simulink library "Scope_new"  (R2017b)
settings: Solver=VariableStepAuto  StartTime=0.0  StopTime=10.0  RelTol=1e-3
undefined symbols (not defined in the file): cal, CycLength, CycNmb, Engine, ess, gb, StopIndex
libraries: simulink x8, EC2_libraries x2
settings Model: Creator=Lyu19  LastModifiedBy=Lyu19

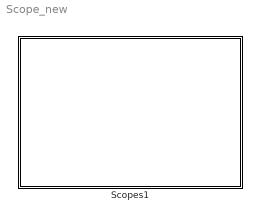
== system Scope_new ==
  Scopes1 : Subsystem
      mask Display: image('Images/Scope.jpg')

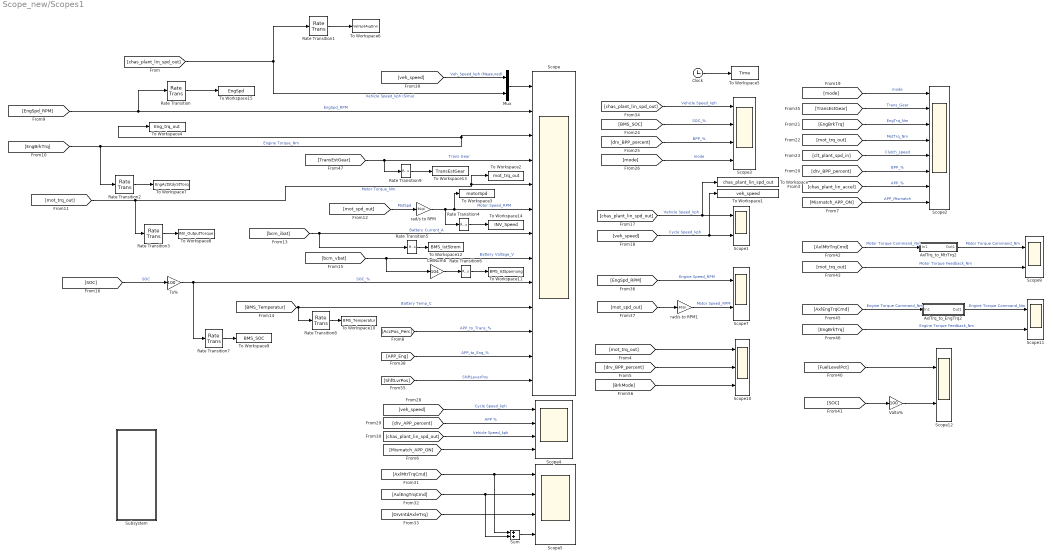
== system Scope_new/Scopes1 ==
  AxlTrq_to_EngTrq2 : Subsystem
  AxlTrq_to_MtrTrq2 : Subsystem
  CellNumb : Gain  Gain=104
  Clock : Clock
      settings: Decimation=WORKSPACE_DECIMATION
  Mux : Mux  Inputs=2
  Rate Transition{,1..9} (10 alike) : RateTransition  OutPortSampleTime=1
  Scope : Scope  NumInputPorts=13
  Scope{1,7,9,11..12} (5 alike) : Scope  NumInputPorts=2
  Scope10 : Scope  NumInputPorts=3
  Scope2 : Scope  NumInputPorts=8
  Scope3 : Scope  NumInputPorts=4
  Scope4 : Scope  NumInputPorts=4
  Scope5 : Scope  NumInputPorts=4
  Subsystem : Subsystem
  Sum : Sum
  To Workspace : ToWorkspace  VariableName=chas_plant_lin_spd_out  SampleTime=-1
  To Workspace1 : ToWorkspace  VariableName=veh_speed  SampleTime=-1
  To Workspace10 : ToWorkspace  VariableName=BMS_Temperatur  SampleTime=-1
  To Workspace11 : ToWorkspace  VariableName=BMS_IstSpannung  SampleTime=-1
  To Workspace12 : ToWorkspace  VariableName=BMS_IstStrom  SampleTime=-1
  To Workspace13 : ToWorkspace  VariableName=TransEstGear  SampleTime=-1
  To Workspace14 : ToWorkspace  VariableName=INV_Speed  SampleTime=-1
  To Workspace15 : ToWorkspace  VariableName=EngSpd  SampleTime=-1
  To Workspace2 : ToWorkspace  VariableName=mot_trq_out  SampleTime=-1
  To Workspace3 : ToWorkspace  VariableName=motorSpd  SampleTime=-1
  To Workspace4 : ToWorkspace  VariableName=Eng_trq_out  SampleTime=-1
  To Workspace5 : ToWorkspace  VariableName=Time  SampleTime=-1
      settings: Decimation=WORKSPACE_DECIMATION
  To Workspace6 : ToWorkspace  VariableName=VehSpdAvgDrvn  SampleTime=-1
  To Workspace7 : ToWorkspace  VariableName=EngActStdyStTorq  SampleTime=-1
  To Workspace8 : ToWorkspace  VariableName=INV_OutputTorque  SampleTime=-1
  To Workspace9 : ToWorkspace  VariableName=BMS_SOC  SampleTime=-1
  To% : Gain  Gain=100
  Valto% : Gain  Gain=100
  rad/s to RPM : Gain  Gain=30/pi
  rad/s to RPM1 : Gain  Gain=30/pi
  wires:
  [chas_plant_lin_spd_out] -> Rate Transition1/1, Mux/2  "Vehicle Speed_kph (Simu)"
  [EngSpd_RPM] -> Rate Transition/1, Scope/2  "EngSpd_RPM"
  [EngBrkTrq] -> Rate Transition2/1, Scope/3, To Workspace4/1  "Engine Torque_Nm"
  [mot_spd_out] -> rad/s to RPM/1  "MotSpd"
  [BMS_Temperatur] -> Rate Transition8/1, Scope/10  "Battery Temp_C"
  rad/s to RPM/1 -> Rate Transition4/1, To Workspace3/1, Scope/6  "Motor Speed_RPM"
  [mot_trq_out] -> Rate Transition3/1, To Workspace2/1, Scope/5  "Motor Torque_Nm"
  To%/1 -> Rate Transition7/1, Scope/9  "SOC_%"
  [TransEstGear] -> Rate Transition9/1, Scope/4  "Trans Gear"
  [bcm_ibat] -> Rate Transition5/1, Scope/7  "Battery Current_A"
  [chas_plant_lin_spd_out] -> Scope3/1  "Vehicle Speed_kph"
  [BMS_SOC] -> Scope3/2  "SOC_%"
  [drv_BPP_percent] -> Scope3/3  "BPP_%"
  [mode] -> Scope3/4  "mode"
  [chas_plant_lin_spd_out] -> To Workspace/1, Scope1/1  "Vehicle Speed_kph"
  [veh_speed] -> To Workspace1/1, Scope1/2  "Cycle Speed_kph"
  [mode] -> Scope2/1  "mode"
  [EngBrkTrq] -> Scope2/3  "EngTrq_Nm"
  [mot_trq_out] -> Scope2/4  "MotTrq_Nm"
  [clt_plant_spd_in] -> Scope2/5  "Clutch_speed"
  [EngSpd_RPM] -> Scope7/1  "Engine Speed_RPM"
  [mot_spd_out] -> rad/s to RPM1/1
  rad/s to RPM1/1 -> Scope7/2  "Motor Speed_RPM"
  [veh_speed] -> Scope4/1  "Cycle Speed_kph"
  [drv_APP_percent] -> Scope4/2  "APP %"
  [chas_plant_lin_spd_out] -> Scope4/3  "Vehicle Speed_kph"
  [AxlMtrTrqCmd] -> Sum/1, Scope5/1
  [AxlEngTrqCmd] -> Sum/2, Scope5/2
  [DrvIntdAxleTrq] -> Scope5/3
  Sum/1 -> Scope5/4
  [AxlMtrTrqCmd] -> AxlTrq_to_MtrTrq2/1(In1)  "Motor Torque Command_Nm"
  [mot_trq_out] -> Scope9/2  "Motor Torque Feedback_Nm"
  [AxlEngTrqCmd] -> AxlTrq_to_EngTrq2/1(In1)  "Engine Torque Command_Nm"
  [EngBrkTrq] -> Scope11/2  "Engine Torque Feedback_Nm"
  [TransEstGear] -> Scope2/2  "Trans_Gear"
  [drv_BPP_percent] -> Scope2/6  "BPP_%"
  [chas_plant_lin_accel] -> Scope2/7  "APP_%"
  AxlTrq_to_MtrTrq2/1(Out1) -> Scope9/1  "Motor Torque Command_Nm"
  AxlTrq_to_EngTrq2/1(Out1) -> Scope11/1  "Engine Torque Command_Nm"
  [bcm_vbat] -> Scope/8, CellNumb/1  "Battery Voltage_V"
  [Mismatch_APP_ON] -> Scope4/4
  [Mismatch_APP_ON] -> Scope2/8  "APP_Mismatch"
  [SOC] -> To%/1  "SOC"
  [AccPos_Perc] -> Scope/11  "APP_to_Trans_%"
  [APP_Eng] -> Scope/12  "APP_to_Eng_%"
  Mux/1 -> Scope/1
  [veh_speed] -> Mux/1  "Veh_Speed_kph (Measured)"
  Clock/1 -> To Workspace5/1
  [FuelLevelPct] -> Scope12/1
  [SOC] -> Valto%/1
  Valto%/1 -> Scope12/2
  [ShftLvrPos] -> Scope/13  "ShiftLeverPos"
  [mot_trq_out] -> Scope10/1
  [drv_BPP_percent] -> Scope10/2
  [BrkMode] -> Scope10/3
  CellNumb/1 -> Rate Transition6/1
  Rate Transition/1 -> To Workspace15/1
  Rate Transition1/1 -> To Workspace6/1
  Rate Transition2/1 -> To Workspace7/1
  Rate Transition3/1 -> To Workspace8/1
  Rate Transition4/1 -> To Workspace14/1
  Rate Transition5/1 -> To Workspace12/1
  Rate Transition6/1 -> To Workspace11/1
  Rate Transition7/1 -> To Workspace9/1
  Rate Transition8/1 -> To Workspace10/1
  Rate Transition9/1 -> To Workspace13/1

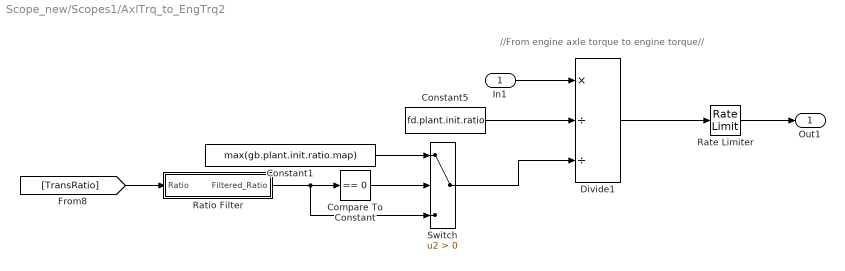
== system Scope_new/Scopes1/AxlTrq_to_EngTrq2 ==
  note: //From engine axle torque to engine torque//
  In1 : Inport
  Compare To Constant : simulink/Logic and Bit Operations/Compare To Constant  relop===  const=0  OutDataTypeStr=boolean
  Constant1 : Constant  Value=max(gb.plant.init.ratio.map)
  Constant5 : Constant  Value=fd.plant.init.ratio
  Divide1 : Product  Inputs=*//
  Rate Limiter : RateLimiter  RisingSlewLimit=Engine.trq_uprate  FallingSlewLimit=Engine.trq_derate
  Ratio Filter : Subsystem
  Switch : Switch  Criteria=u2 > Threshold
  Out1 : Outport
  wires:
  In1/1 -> Divide1/1
  Constant5/1 -> Divide1/2
  Divide1/1 -> Rate Limiter/1
  [TransRatio] -> Ratio Filter/1(Ratio)
  Compare To Constant/1 -> Switch/2
  Constant1/1 -> Switch/1
  Switch/1 -> Divide1/3
  Rate Limiter/1 -> Out1/1
  Ratio Filter/1(Filtered_Ratio) -> Switch/3, Compare To Constant/1

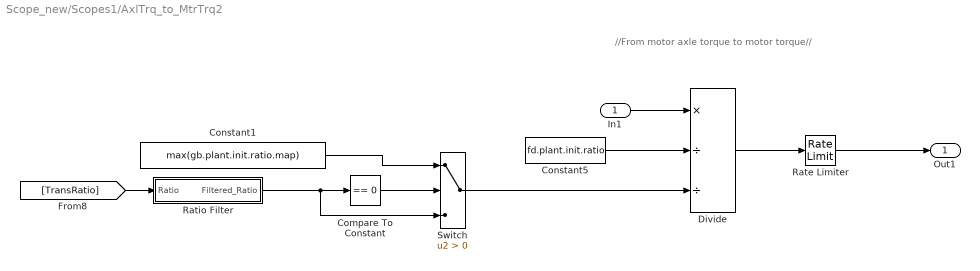
== system Scope_new/Scopes1/AxlTrq_to_MtrTrq2 ==
  note: //From motor axle torque to motor torque//
  In1 : Inport
  Compare To Constant : simulink/Logic and Bit Operations/Compare To Constant  relop===  const=0  OutDataTypeStr=boolean
  Constant1 : Constant  Value=max(gb.plant.init.ratio.map)
  Constant5 : Constant  Value=fd.plant.init.ratio
  Divide : Product  Inputs=*//
  Rate Limiter : RateLimiter  RisingSlewLimit=mcu.plant.init.trq_uprate  FallingSlewLimit=mcu.plant.init.trq_derate
  Ratio Filter : Subsystem
  Switch : Switch  Criteria=u2 > Threshold
  Out1 : Outport
  wires:
  In1/1 -> Divide/1
  Constant5/1 -> Divide/2
  Divide/1 -> Rate Limiter/1
  [TransRatio] -> Ratio Filter/1(Ratio)
  Compare To Constant/1 -> Switch/2
  Constant1/1 -> Switch/1
  Rate Limiter/1 -> Out1/1
  Switch/1 -> Divide/3
  Ratio Filter/1(Filtered_Ratio) -> Switch/3, Compare To Constant/1

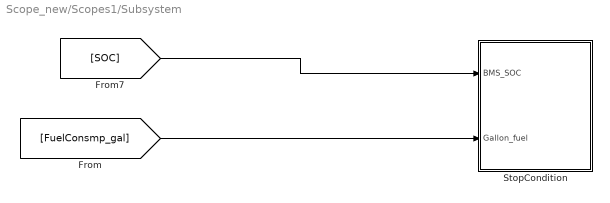
== system Scope_new/Scopes1/Subsystem ==
  "StopCondition " : Subsystem
  wires:
  [SOC] -> "StopCondition "/1(BMS_SOC)
  [FuelConsmp_gal] -> "StopCondition "/2(Gallon_fuel)

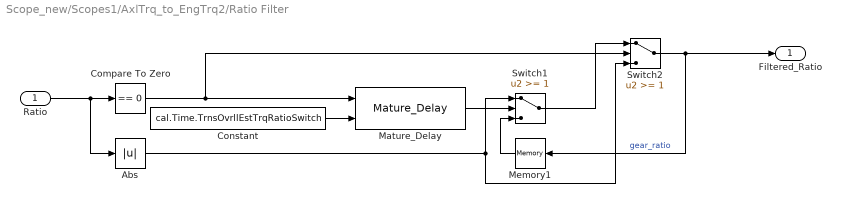
== system Scope_new/Scopes1/AxlTrq_to_EngTrq2/Ratio Filter ==
  Ratio : Inport
  Abs : Abs
  Compare To Zero : simulink/Logic and Bit Operations/Compare To Zero  relop===  OutDataTypeStr=boolean
  Constant : Constant  Value=cal.Time.TrnsOvrllEstTrqRatioSwitch
  Mature_Delay : EC2_libraries/Mature_Delay
      settings: SourceProductName=The database C:\Users\vrajm\AppData\Roaming\MathWorks\MATLAB\R2017b\slblocks_master.db is locked, or a table in the database is locked. (database is locked)
  Memory1 : Memory  InitialCondition=1
  Switch1 : Switch  Threshold=1
  Switch2 : Switch  Threshold=1
  Filtered_Ratio : Outport
  wires:
  Ratio/1 -> Compare To Zero/1, Abs/1
  Compare To Zero/1 -> Mature_Delay/1, Switch2/2
  Abs/1 -> Switch1/1, Switch2/3
  Switch1/1 -> Switch2/1
  Constant/1 -> Mature_Delay/2
  Mature_Delay/1 -> Switch1/2
  Memory1/1 -> Switch1/3
  Switch2/1 -> Filtered_Ratio/1, Memory1/1  "gear_ratio"

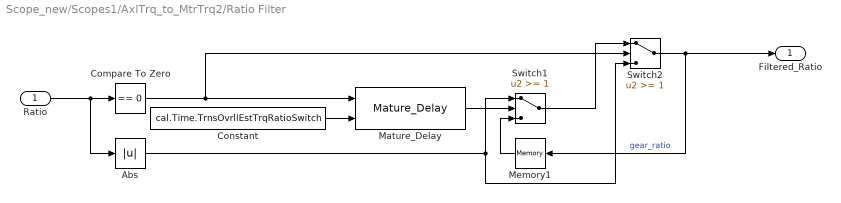
== system Scope_new/Scopes1/AxlTrq_to_MtrTrq2/Ratio Filter ==
  Ratio : Inport
  Abs : Abs
  Compare To Zero : simulink/Logic and Bit Operations/Compare To Zero  relop===  OutDataTypeStr=boolean
  Constant : Constant  Value=cal.Time.TrnsOvrllEstTrqRatioSwitch
  Mature_Delay : EC2_libraries/Mature_Delay
      settings: SourceProductName=The database C:\Users\vrajm\AppData\Roaming\MathWorks\MATLAB\R2017b\slblocks_master.db is locked, or a table in the database is locked. (database is locked)
  Memory1 : Memory  InitialCondition=1
  Switch1 : Switch  Threshold=1
  Switch2 : Switch  Threshold=1
  Filtered_Ratio : Outport
  wires:
  Ratio/1 -> Compare To Zero/1, Abs/1
  Compare To Zero/1 -> Mature_Delay/1, Switch2/2
  Abs/1 -> Switch1/1, Switch2/3
  Switch1/1 -> Switch2/1
  Constant/1 -> Mature_Delay/2
  Mature_Delay/1 -> Switch1/2
  Memory1/1 -> Switch1/3
  Switch2/1 -> Filtered_Ratio/1, Memory1/1  "gear_ratio"

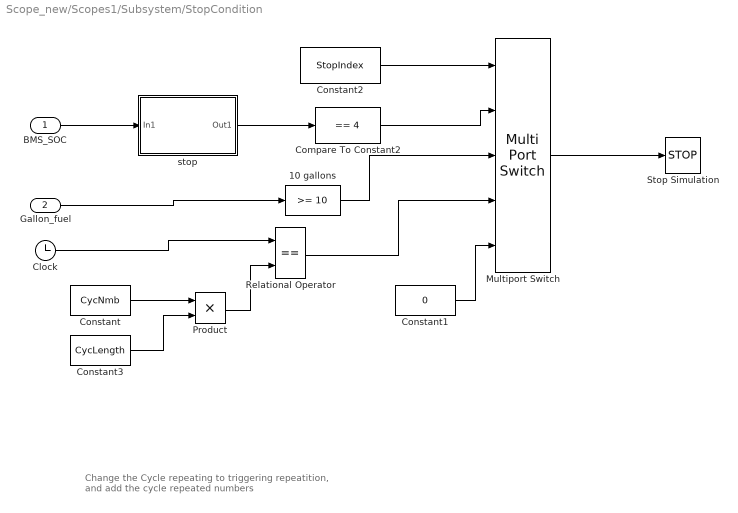
== system Scope_new/Scopes1/Subsystem/StopCondition  ==
  note: Change the Cycle repeating to triggering repeatition,
      | and add the cycle repeated numbers
  BMS_SOC : Inport
  Gallon_fuel : Inport  Port=2
  10 gallons : simulink/Logic and Bit Operations/Compare To Constant  relop=>=  const=10  OutDataTypeStr=boolean
  Clock : Clock
  Compare To Constant2 : simulink/Logic and Bit Operations/Compare To Constant  relop===  const=4  OutDataTypeStr=boolean
  Constant : Constant  Value=CycNmb
  Constant1 : Constant  Value=0
  Constant2 : Constant  Value=StopIndex
  Constant3 : Constant  Value=CycLength
  Multiport Switch : MultiPortSwitch  Inputs=4
  Product : Product
  Relational Operator : RelationalOperator  Operator===  OutDataTypeStr=boolean  RndMeth=Simplest
  Stop Simulation : Stop
  "stop " : Subsystem
  wires:
  Clock/1 -> Relational Operator/1
  Multiport Switch/1 -> Stop Simulation/1
  Constant2/1 -> Multiport Switch/1
  BMS_SOC/1 -> "stop "/1(In1)
  10 gallons/1 -> Multiport Switch/3
  "stop "/1(Out1) -> Compare To Constant2/1
  Compare To Constant2/1 -> Multiport Switch/2
  Gallon_fuel/1 -> 10 gallons/1
  Constant/1 -> Product/1
  Relational Operator/1 -> Multiport Switch/4
  Constant1/1 -> Multiport Switch/5
  Product/1 -> Relational Operator/2
  Constant3/1 -> Product/2

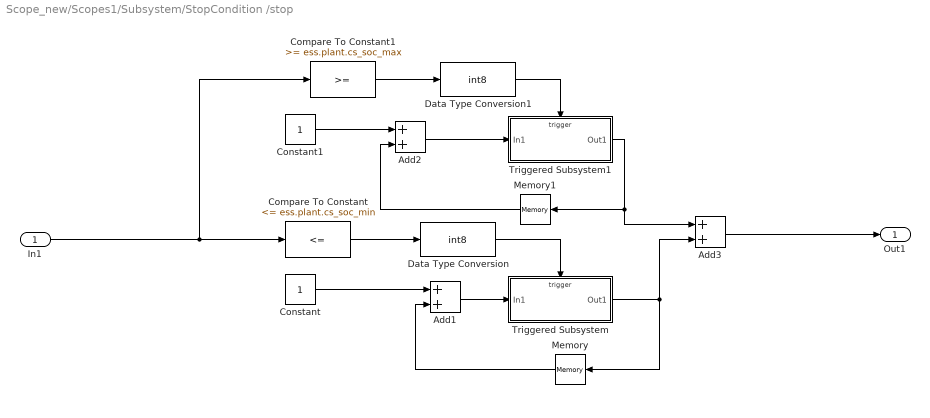
== system Scope_new/Scopes1/Subsystem/StopCondition /stop  ==
  In1 : Inport
  Add1 : Sum
  Add2 : Sum
  Add3 : Sum
  Compare To Constant : simulink/Logic and Bit Operations/Compare To Constant  relop=<=  const=ess.plant.cs_soc_min  OutDataTypeStr=boolean
  Compare To Constant1 : simulink/Logic and Bit Operations/Compare To Constant  relop=>=  const=ess.plant.cs_soc_max  OutDataTypeStr=boolean
  Constant : Constant
  Constant1 : Constant
  Data Type Conversion : DataTypeConversion  OutDataTypeStr=int8
  Data Type Conversion1 : DataTypeConversion  OutDataTypeStr=int8
  Memory : Memory
  Memory1 : Memory
  Triggered Subsystem : Subsystem  TreatAsAtomicUnit=on
  Triggered Subsystem1 : Subsystem  TreatAsAtomicUnit=on
  Out1 : Outport
  wires:
  Compare To Constant/1 -> Data Type Conversion/1
  Data Type Conversion1/1 -> Triggered Subsystem1/Trigger
  Add3/1 -> Out1/1
  Add2/1 -> Triggered Subsystem1/1(In1)
  Triggered Subsystem1/1(Out1) -> Add3/1, Memory1/1
  Constant1/1 -> Add2/1
  In1/1 -> Compare To Constant1/1, Compare To Constant/1
  Compare To Constant1/1 -> Data Type Conversion1/1
  Memory1/1 -> Add2/2
  Memory/1 -> Add1/2
  Data Type Conversion/1 -> Triggered Subsystem/Trigger
  Add1/1 -> Triggered Subsystem/1(In1)
  Constant/1 -> Add1/1
  Triggered Subsystem/1(Out1) -> Add3/2, Memory/1

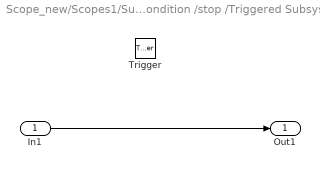
== system Scope_new/Scopes1/Subsystem/StopCondition /stop /Triggered Subsystem ==
  In1 : Inport
  Trigger : TriggerPort  VariantControl=Variant
  Out1 : Outport
  wires:
  In1/1 -> Out1/1

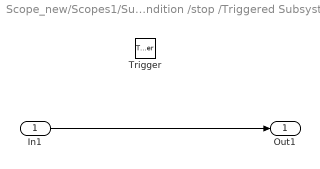
== system Scope_new/Scopes1/Subsystem/StopCondition /stop /Triggered Subsystem1 ==
  In1 : Inport
  Trigger : TriggerPort  VariantControl=Variant
  Out1 : Outport
  wires:
  In1/1 -> Out1/1
